simulink model "PARED_RT_SFR"  (R2015a)
settings: Solver=ode4  SolverMode=SingleTasking  StartTime=0.0  StopTime=inf  FixedStep=ts  RelTol=1e-3
InitFcn:
  | tc=ts;
values from neighbouring files (symbols this model uses):
  Kcd = place(matAd,matBud,polosd_lc)    [CONTROL_SEGWAY_BASE_PASADO.m]    (also in analiza_robustez_SFR.m = Kcd.*repmat(Ybase',n_u,1).*repmat(1../Ubase,1,n_y); diseno_control_integral.m = Ka(1, 1:3); diseno_regulador.m = place(Ad, Bd, polosd_lc); maestro.m = place (matAd , matBd , polosd_lc))
  Kcd_pared = acker(matAdp,matBdp(:,1),polosd_lc_pared)    [CONTROL_SEGWAY_BASE_PASADO.m]    (also in diseno_control_seguimiento_pared.m = place(Adp, Bdp(:,1), polosd_lcp))
  Kid = Kad(:,4)    [CONTROL_SEGWAY_BASE_PASADO.m]    (also in diseno_control_integral.m = Ka(1,4))
  R = 81.6e-3/2    (= 0.0408)    [CONTROL_SEGWAY.m]    (also in CONTROL_SEGWAY_BASE_PASADO.m; diseno_control_integral.m; diseno_control_pid.m; diseno_regulador.m)
  sound_freq = 440    [CONTROL_SEGWAY.m]    (also in CONTROL_SEGWAY_BASE_PASADO.m; diseno_control_integral.m; diseno_control_pid.m; diseno_regulador.m)
  time_start = 1    [CONTROL_SEGWAY.m]    (also in CONTROL_SEGWAY_BASE_PASADO.m; diseno_control_integral.m; diseno_control_pid.m; diseno_regulador.m)
  ts = 5e-3    (= 0.005)    [CONTROL_SEGWAY.m]    (also in CONTROL_SEGWAY_BASE_PASADO.m = 0.1; analiza_robustez_SFR.m = Pss_d.Ts; diseno_control_integral.m; diseno_control_pid.m)
  W = 0.15    [CONTROL_SEGWAY.m]    (also in CONTROL_SEGWAY_BASE_PASADO.m; diseno_control_integral.m; diseno_control_pid.m; diseno_regulador.m)
  Wfc = 0.98    [CONTROL_SEGWAY.m]    (also in CONTROL_SEGWAY_BASE_PASADO.m; diseno_control_integral.m; diseno_control_pid.m; diseno_regulador.m)
undefined symbols (not defined in the file or in its folder): D, D1, D2, Fi, gr, mm, rw, th
undefined symbols (not defined in the file): alfa1, gyro0
libraries: legonxtlib x22, simulink x4
settings Model: SimulationMode=external  ExtModeTrigDuration=2  Creator=jrperez  LastModifiedBy=zamora
settings DataIOCC: SignalLoggingSaveFormat=ModelDataLogs
settings OptimizationCC: ExpressionDepthLimit=2147483647  OptimizeModelRefInitCode=on  LifeSpan=1
settings DebuggingCC: UnderspecifiedInitializationDetection=Classic  MergeDetectMultiDrivingBlocksExec=none  ParameterPrecisionLossMsg=none  FcnCallInpInsideContextMsg=EnableAllAsWarning  StateNameClashWarn=warning
settings HardwareCC: ProdLargestAtomicInteger=Long  ProdLargestAtomicFloat=Float  ProdEndianess=LittleEndian  ProdHWDeviceType=ARM Compatible->ARM 7
settings RTWCC: SystemTargetFile=realtime.tlc  GenerateMakefile=off  TemplateMakefile=realtime.tmf  Description=Real-Time Toolbox  RTWVerbose=off
settings CodeAppCC: CustomSymbolStrType=$N$R$M  InternalIdentifier=Classic
settings ERTTargetCC: CombineOutputUpdateFcns=off  ExtMode=on  ExtModeTransport=2  ExtModeMexFile=ext_serial_win32_comm_no_acks_rtt  ExtModeMexArgs=0 10 9600 30  InlinedParameterPlacement=Hierarchical  ERTSrcFileBannerTemplate=realtime_code_template.cgt  ERTHdrFileBannerTemplate=realtime_code_template.cgt  ERTDataSrcFileTemplate=realtime_code_template.cgt  ERTDataHdrFileTemplate=realtime_code_template.cgt  ERTCustomFileTemplate=realtime_file_process.tlc

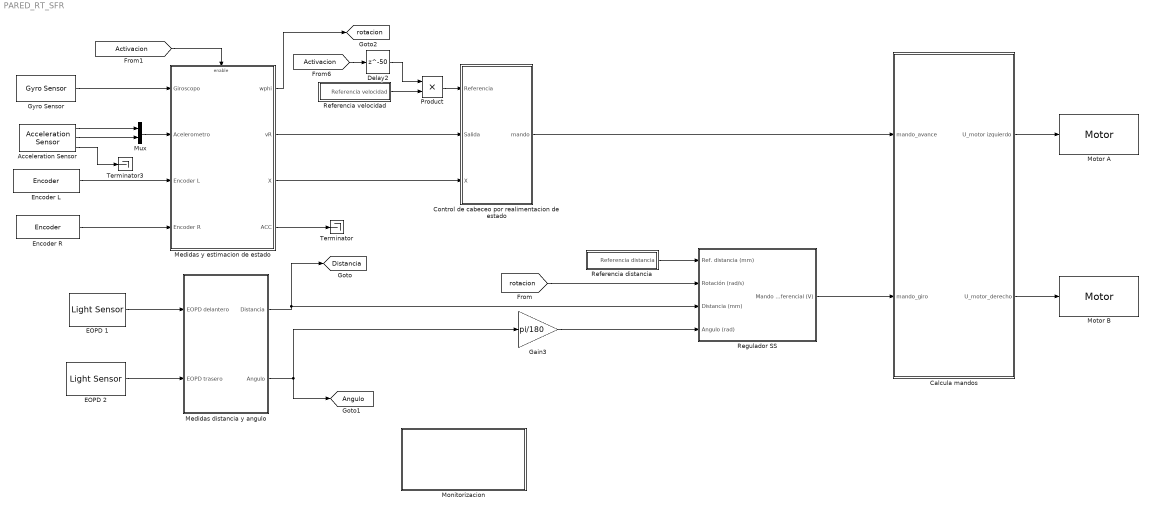
== system PARED_RT_SFR ==
  Acceleration Sensor : legonxtlib/Acceleration Sensor  portNumber=2  sampleTime=ts  blockPlatform=LegoMindstormsNXT
  Calcula mandos : Subsystem
  Control de cabeceo por realimentacion de estado : Subsystem
  Delay2 : Delay  DelayLength=50
  EOPD 1 : legonxtlib/Light Sensor  portNumber=1  outputMode=Raw A/D (1023 - 0)  lightOn=on  sampleTime=ts  blockPlatform=LegoMindstormsNXT
  EOPD 2 : legonxtlib/Light Sensor  portNumber=4  outputMode=Raw A/D (1023 - 0)  lightOn=on  sampleTime=ts  blockPlatform=LegoMindstormsNXT
  Encoder L : legonxtlib/Encoder  portNumber=B  opMode=No reset  sampleTime=ts  blockPlatform=LegoMindstormsNXT
  Encoder R : legonxtlib/Encoder  portNumber=C  opMode=No reset  sampleTime=ts  blockPlatform=LegoMindstormsNXT
  Gain3 : Gain  Gain=pi/180
  Gyro Sensor : legonxtlib/Gyro Sensor  portNumber=3  outputMode=Raw A/D (0 - 1023)  offset=600  sampleTime=ts  blockPlatform=LegoMindstormsNXT
  Medidas distancia y angulo : Subsystem
  Medidas y estimacion de estado : Subsystem
  Monitorizacion : Subsystem
  Motor A : legonxtlib/Motor  sportNumber=B  sstopAction=Brake  blockPlatform=LegoMindstormsNXT
  Motor B : legonxtlib/Motor  sportNumber=C  sstopAction=Brake  blockPlatform=LegoMindstormsNXT
  Mux : Mux  Inputs=2
  Product : Product  RndMeth=Zero
  Referencia distancia : Subsystem
  Referencia velocidad : Subsystem
  Regulador SS : Subsystem
  Terminator : Terminator
  Terminator3 : Terminator
  tag scope: Angulo=global, Distancia=global, rotacion=global
  wires:
  Calcula mandos/1(U_motor izquierdo) -> Motor A/1
  Calcula mandos/2(U_motor_derecho) -> Motor B/1
  Control de cabeceo por realimentacion de estado/1(mando) -> Calcula mandos/1(mando_avance)
  EOPD 1/1 -> Medidas distancia y angulo/1(EOPD delantero)
  EOPD 2/1 -> Medidas distancia y angulo/2(EOPD trasero)
  Medidas distancia y angulo/1(Distancia) -> Regulador SS/3(Distancia (mm)), [Distancia]
  Medidas y estimacion de estado/4(ACC) -> Terminator/1
  [Activacion] -> Delay2/1
  Product/1 -> Control de cabeceo por realimentacion de estado/1(Referencia)
  Referencia velocidad/1(Referencia velocidad) -> Product/2
  Delay2/1 -> Product/1
  Gyro Sensor/1 -> Medidas y estimacion de estado/1(Giroscopo)
  Encoder L/1 -> Medidas y estimacion de estado/3(Encoder L)
  Encoder R/1 -> Medidas y estimacion de estado/4(Encoder R)
  Acceleration Sensor/3 -> Terminator3/1
  Acceleration Sensor/1 -> Mux/1
  Acceleration Sensor/2 -> Mux/2
  Mux/1 -> Medidas y estimacion de estado/2(Acelerometro)
  Medidas y estimacion de estado/2(vR) -> Control de cabeceo por realimentacion de estado/2(Salida)
  Medidas y estimacion de estado/3(X) -> Control de cabeceo por realimentacion de estado/3(X)
  [Activacion] -> Medidas y estimacion de estado/Enable
  Medidas y estimacion de estado/1(wphi) -> [rotacion]
  Medidas distancia y angulo/2(Angulo) -> [Angulo], Gain3/1
  [rotacion] -> Regulador SS/2(Rotación (rad/s))
  Referencia distancia/1(Referencia distancia) -> Regulador SS/1(Ref. distancia (mm))
  Gain3/1 -> Regulador SS/4(Angulo (rad))
  Regulador SS/1(Mando diferencial (V)) -> Calcula mandos/2(mando_giro)

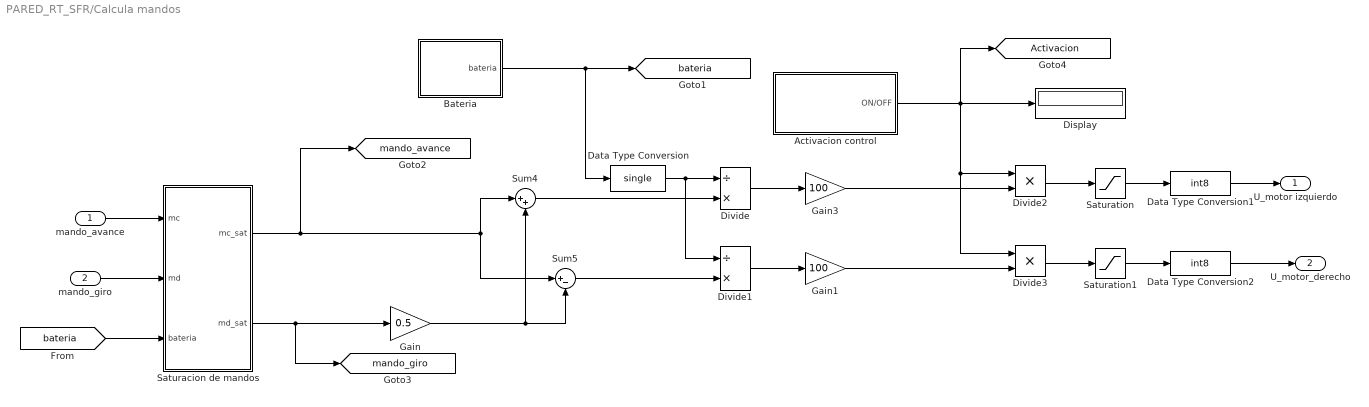
== system PARED_RT_SFR/Calcula mandos ==
  mando_avance : Inport
  mando_giro : Inport  Port=2
  Activacion control : Subsystem
  Bateria : Subsystem
  Data Type Conversion : DataTypeConversion  OutDataTypeStr=single  SampleTime=ts
  Data Type Conversion1 : DataTypeConversion  OutDataTypeStr=int8
  Data Type Conversion2 : DataTypeConversion  OutDataTypeStr=int8
  Display : Display
  Divide : Product  Inputs=/*  SampleTime=ts
  Divide1 : Product  Inputs=/*  SampleTime=ts
  Divide2 : Product  SampleTime=ts
  Divide3 : Product  SampleTime=ts
  Gain : Gain  Gain=0.5  OutDataTypeStr=single
  Gain1 : Gain  Gain=100
  Gain3 : Gain  Gain=100
  Saturacion de mandos : Subsystem
  Saturation : Saturate  UpperLimit=100  LowerLimit=-100
  Saturation1 : Saturate  UpperLimit=100  LowerLimit=-100
  Sum4 : Sum  Inputs=|++
  Sum5 : Sum  Inputs=|+-
  U_motor izquierdo : Outport
  U_motor_derecho : Outport  Port=2
  tag scope: Activacion=global, bateria=global, mando_avance=global, mando_giro=global
  wires:
  Divide/1 -> Gain3/1
  Sum4/1 -> Divide/2
  Gain3/1 -> Divide2/2
  Divide1/1 -> Gain1/1
  Sum5/1 -> Divide1/2
  Saturacion de mandos/1(mc_sat) -> Sum4/1, Sum5/1, [mando_avance]
  Saturacion de mandos/2(md_sat) -> [mando_giro], Gain/1
  Bateria/1(bateria) -> Data Type Conversion/1, [bateria]
  Divide2/1 -> Saturation/1
  Divide3/1 -> Saturation1/1
  Data Type Conversion1/1 -> U_motor izquierdo/1
  Data Type Conversion2/1 -> U_motor_derecho/1
  Data Type Conversion/1 -> Divide/1, Divide1/1
  Gain1/1 -> Divide3/2
  Saturation/1 -> Data Type Conversion1/1
  Saturation1/1 -> Data Type Conversion2/1
  [bateria] -> Saturacion de mandos/3(bateria)
  mando_avance/1 -> Saturacion de mandos/1(mc)
  mando_giro/1 -> Saturacion de mandos/2(md)
  Activacion control/1(ON/OFF) -> Display/1, [Activacion], Divide2/1, Divide3/1
  Gain/1 -> Sum4/2, Sum5/2

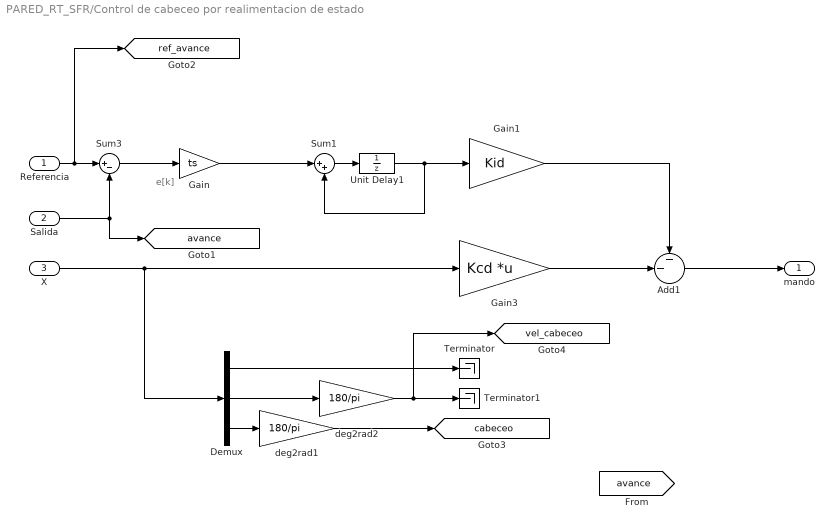
== system PARED_RT_SFR/Control de cabeceo por realimentacion de estado ==
  note: e[k]
  Referencia : Inport
  Salida : Inport  Port=2
  X : Inport  Port=3  SampleTime=ts
  Add1 : Sum  Inputs=--|
  Demux : Demux  Outputs=3
  Gain : Gain  Gain=ts  RndMeth=Simplest  OutDataTypeStr=Inherit: Same as input
  Gain1 : Gain  Gain=Kid  RndMeth=Simplest  SaturateOnIntegerOverflow=on  OutDataTypeStr=Inherit: Same as input  ParamDataTypeStr=Inherit: Same as input
  Gain3 : Gain  Gain=Kcd  Multiplication=Matrix(K*u) (u vector)  SaturateOnIntegerOverflow=on  OutDataTypeStr=Inherit: Same as input  ParamDataTypeStr=Inherit: Same as input
  Sum1 : Sum  Inputs=|++  AccumDataTypeStr=single
  Sum3 : Sum  Inputs=|+-  AccumDataTypeStr=single
  Terminator : Terminator
  Terminator1 : Terminator
  Unit Delay1 : UnitDelay  SampleTime=-1
  deg2rad1 : Gain  Gain=180/pi  OutDataTypeStr=Inherit: Same as input  ParamDataTypeStr=Inherit: Same as input
  deg2rad2 : Gain  Gain=180/pi  OutDataTypeStr=Inherit: Same as input  ParamDataTypeStr=Inherit: Same as input
  mando : Outport
  tag scope: avance=global, cabeceo=global, ref_avance=global, vel_cabeceo=global
  wires:
  Add1/1 -> mando/1
  Unit Delay1/1 -> Gain1/1, Sum1/2
  Referencia/1 -> Sum3/1, [ref_avance]
  Salida/1 -> Sum3/2, [avance]
  Sum3/1 -> Gain/1
  Sum1/1 -> Unit Delay1/1
  Gain1/1 -> Add1/1
  Gain3/1 -> Add1/2
  X/1 -> Gain3/1, Demux/1
  Demux/1 -> Terminator/1
  Demux/2 -> deg2rad2/1
  Demux/3 -> deg2rad1/1
  deg2rad1/1 -> [cabeceo]
  Gain/1 -> Sum1/1
  deg2rad2/1 -> [vel_cabeceo], Terminator1/1

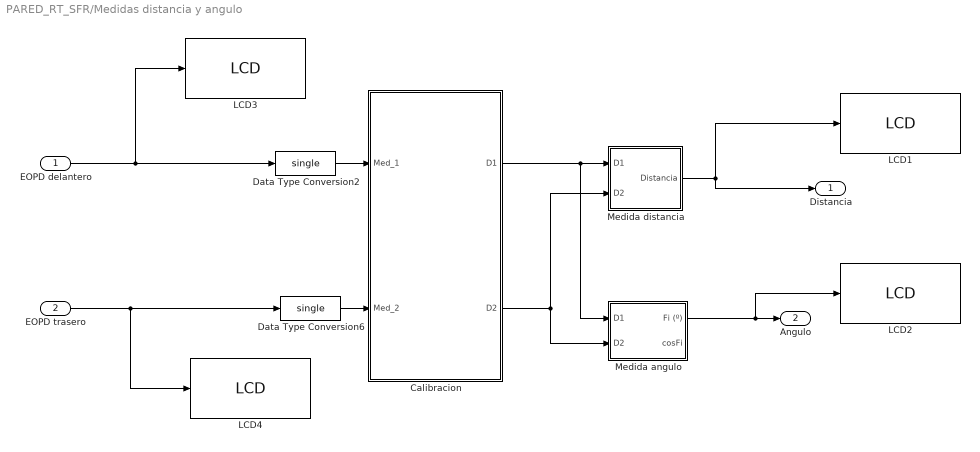
== system PARED_RT_SFR/Medidas distancia y angulo ==
  EOPD delantero : Inport
  EOPD trasero : Inport  Port=2
  "Calibracion " : Subsystem  mask{distNear=50, distFar=100, eopdNear_1=725, eopdNear_2=732, eopdFar_1=917, eopdFar_2=922, ts=ts}
      mask prompts: distNear "Distancia cercana (mm)"; distFar "Distancia lejana (mm)"; eopdNear_1 "Medida D1 cercana (raw)"; eopdNear_2 "Medida D2  cercana (raw)"; eopdFar_1 "Medida D1 lejana (raw)"; eopdFar_2 "Medida D2 lejana (raw)"; ts "Período de muestreo"
      mask init:
      | % Ver justificacion en:
      | % http://www.hitechnic.com/blog/eopd-sensor/eopd-how-to-measure-distance/
  Data Type Conversion2 : DataTypeConversion  OutDataTypeStr=single
  Data Type Conversion6 : DataTypeConversion  OutDataTypeStr=single
  LCD1 : legonxtlib/LCD  slcdStr=D(mm)  slcdLine=1  slcdFormat=Decimal  blockPlatform=LegoMindstormsNXT
  LCD2 : legonxtlib/LCD  slcdStr=Fi(gr)  slcdLine=2  slcdFormat=Decimal  blockPlatform=LegoMindstormsNXT
  LCD3 : legonxtlib/LCD  slcdStr=D1(rw)  slcdLine=3  slcdFormat=Decimal  blockPlatform=LegoMindstormsNXT
  LCD4 : legonxtlib/LCD  slcdStr=D2(rw)  slcdLine=4  slcdFormat=Decimal  blockPlatform=LegoMindstormsNXT
  Medida distancia : Subsystem
  Medida angulo : Subsystem
  Distancia : Outport
  Angulo : Outport  Port=2
  wires:
  Data Type Conversion2/1 -> "Calibracion "/1(Med_1)
  Data Type Conversion6/1 -> "Calibracion "/2(Med_2)
  EOPD delantero/1 -> Data Type Conversion2/1, LCD3/1
  EOPD trasero/1 -> Data Type Conversion6/1, LCD4/1
  "Calibracion "/1(D1) -> Medida distancia/1(D1), Medida angulo/1(D1)
  "Calibracion "/2(D2) -> Medida distancia/2(D2), Medida angulo/2(D2)
  Medida angulo/1(Fi (º)) -> Angulo/1, LCD2/1
  Medida distancia/1(Distancia) -> Distancia/1, LCD1/1

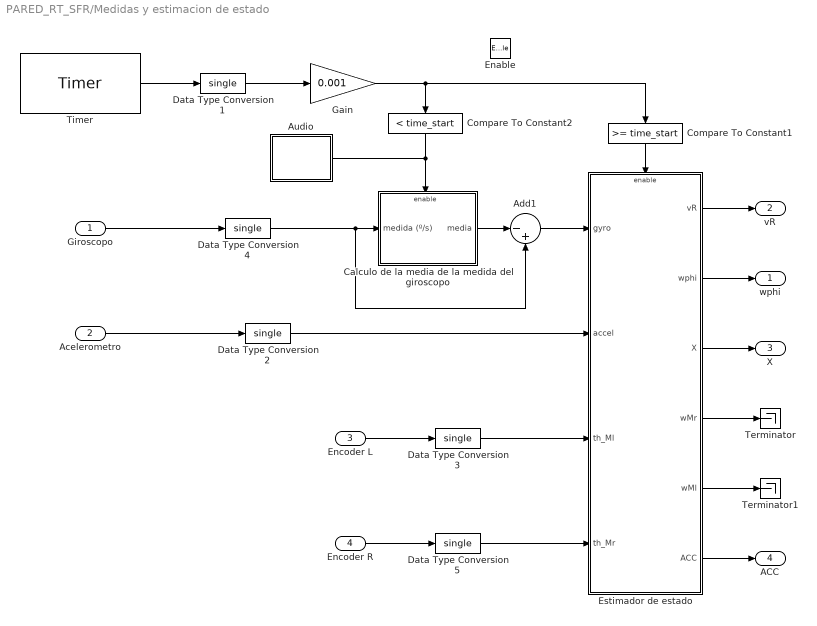
== system PARED_RT_SFR/Medidas y estimacion de estado ==
  Giroscopo : Inport
  Acelerometro : Inport  Port=2
  Encoder L : Inport  Port=3
  Encoder R : Inport  Port=4
  Enable : EnablePort
  Add1 : Sum  Inputs=|-+
  Audio : Subsystem
  Calculo de la media de la medida del giroscopo : Subsystem
  Compare To Constant1 : simulink/Logic and Bit Operations/Compare To Constant  relop=>=  const=time_start  OutDataTypeStr=boolean
  Compare To Constant2 : simulink/Logic and Bit Operations/Compare To Constant  relop=<  const=time_start  OutDataTypeStr=boolean
  Data Type Conversion{1..5} (5 alike) : DataTypeConversion  OutDataTypeStr=single  RndMeth=Simplest
      settings: AttributesFormatString=Round = %<RndMeth>
  Estimador de estado : Subsystem
  Gain : Gain  Gain=0.001
  Terminator : Terminator
  Terminator1 : Terminator
  Timer : legonxtlib/Timer  sampleTime=ts  blockPlatform=LegoMindstormsNXT
  wphi : Outport
  vR : Outport  Port=2
  X : Outport  Port=3
  ACC : Outport  Port=4
  wires:
  Data Type Conversion4/1 -> Calculo de la media de la medida del giroscopo/1(medida (º/s)), Add1/2
  Calculo de la media de la medida del giroscopo/1(media) -> Add1/1
  Giroscopo/1 -> Data Type Conversion4/1
  Compare To Constant2/1 -> Calculo de la media de la medida del giroscopo/Enable, Audio/Enable
  Encoder L/1 -> Data Type Conversion3/1
  Encoder R/1 -> Data Type Conversion5/1
  Add1/1 -> Estimador de estado/1(gyro)
  Data Type Conversion3/1 -> Estimador de estado/3(th_Ml)
  Data Type Conversion5/1 -> Estimador de estado/4(th_Mr)
  Estimador de estado/5(wMl) -> Terminator1/1
  Estimador de estado/4(wMr) -> Terminator/1
  Estimador de estado/1(vR) -> vR/1
  Estimador de estado/2(wphi) -> wphi/1
  Estimador de estado/3(X) -> X/1
  Gain/1 -> Compare To Constant2/1, Compare To Constant1/1
  Timer/1 -> Data Type Conversion1/1
  Compare To Constant1/1 -> Estimador de estado/Enable
  Data Type Conversion1/1 -> Gain/1
  Data Type Conversion2/1 -> Estimador de estado/2(accel)
  Acelerometro/1 -> Data Type Conversion2/1
  Estimador de estado/6(ACC) -> ACC/1

== system PARED_RT_SFR/Monitorizacion ==
  Medidas : Scope
      settings: TimeRange=auto  MaxDataPoints=5000  SaveName=Medidas  YMin=-10  YMax=10  SampleTime=-1  DataFormat=Array
  Mux1 : Mux  Inputs=8
  wires:
  Mux1/1 -> Medidas/1
  [cabeceo] -> Mux1/1
  [vel_cabeceo] -> Mux1/2
  [avance] -> Mux1/3
  [mando_avance] -> Mux1/4
  [Distancia] -> Mux1/5
  [rotacion] -> Mux1/7
  [Angulo] -> Mux1/6
  [mando_giro] -> Mux1/8

== system PARED_RT_SFR/Referencia distancia ==
  ang_ref maximo2 : Constant  Value=100  OutDataTypeStr=single  SampleTime=ts
  Referencia distancia : Outport
  wires:
  ang_ref maximo2/1 -> Referencia distancia/1

== system PARED_RT_SFR/Referencia velocidad ==
  ang_ref maximo2 : Constant  Value=-0.15  OutDataTypeStr=single  SampleTime=ts
  Referencia velocidad : Outport
  wires:
  ang_ref maximo2/1 -> Referencia velocidad/1

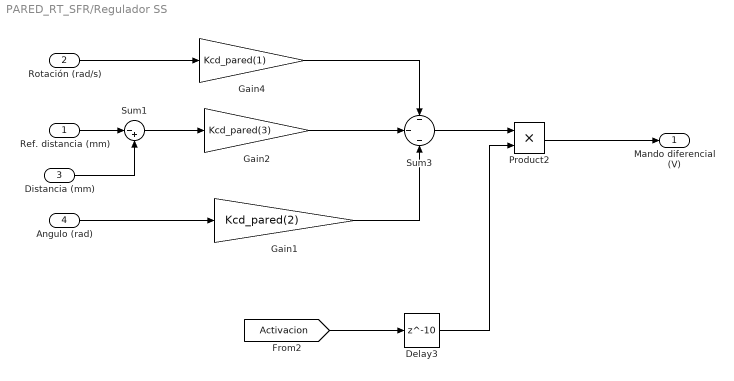
== system PARED_RT_SFR/Regulador SS ==
  Ref. distancia (mm) : Inport
  Rotación (rad/s) : Inport  Port=2
  Distancia (mm) : Inport  Port=3
  Angulo (rad) : Inport  Port=4
  Delay3 : Delay  DelayLength=10
  Gain1 : Gain  Gain=Kcd_pared(2)
  Gain2 : Gain  Gain=Kcd_pared(3)
  Gain4 : Gain  Gain=Kcd_pared(1)
  Product2 : Product  RndMeth=Zero
  Sum1 : Sum  Inputs=|-+
  Sum3 : Sum  Inputs=-|-|-
  Mando diferencial (V) : Outport
  wires:
  Sum1/1 -> Gain2/1
  Sum3/1 -> Product2/1
  Delay3/1 -> Product2/2
  Gain1/1 -> Sum3/3
  Gain4/1 -> Sum3/1
  Rotación (rad/s)/1 -> Gain4/1
  Angulo (rad)/1 -> Gain1/1
  Product2/1 -> Mando diferencial (V)/1
  [Activacion] -> Delay3/1
  Ref. distancia (mm)/1 -> Sum1/1
  Gain2/1 -> Sum3/2
  Distancia (mm)/1 -> Sum1/2

== system PARED_RT_SFR/Calcula mandos/Activacion control ==
  Button : legonxtlib/Button  buttonType=Middle orange  sampleTime=0.1  blockPlatform=LegoMindstormsNXT
  Data Type Conversion : DataTypeConversion  OutDataTypeStr=single
  Saturation : Saturate  UpperLimit=1  LowerLimit=0
  Switch : Switch  Threshold=0.5
  Unit Delay : UnitDelay  SampleTime=0.1
  ON/OFF : Outport
  wires:
  Button/1 -> Data Type Conversion/1
  Switch/1 -> Saturation/1
  Unit Delay/1 -> Switch/3
  Data Type Conversion/1 -> Switch/2, Switch/1
  Saturation/1 -> Unit Delay/1, ON/OFF/1

== system PARED_RT_SFR/Calcula mandos/Bateria ==
  Battery : legonxtlib/Battery  sampleTime=0.1  blockPlatform=LegoMindstormsNXT
  Data Type Conversion : DataTypeConversion  OutDataTypeStr=double
  Data Type Conversion1 : DataTypeConversion  OutDataTypeStr=single
  Gain1 : Gain  Gain=1/5
  Gain6 : Gain  Gain=0.001
  Integrator : Integrator  InitialConditionSource=external
  Sum1 : Sum  Inputs=|+-
  bateria : Outport
  wires:
  Battery/1 -> Data Type Conversion/1
  Data Type Conversion/1 -> Gain6/1
  Sum1/1 -> Gain1/1
  Integrator/1 -> Sum1/2, Data Type Conversion1/1
  Gain6/1 -> Sum1/1, Integrator/2
  Gain1/1 -> Integrator/1
  Data Type Conversion1/1 -> bateria/1

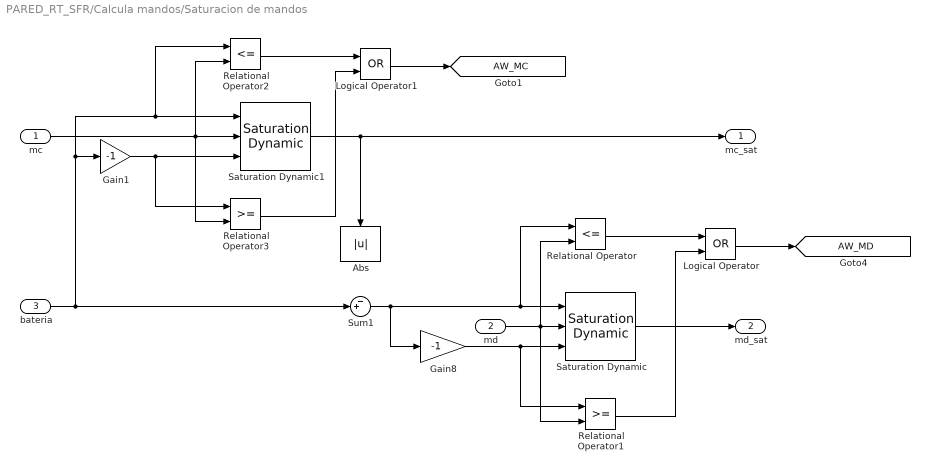
== system PARED_RT_SFR/Calcula mandos/Saturacion de mandos ==
  mc : Inport
  md : Inport  Port=2
  bateria : Inport  Port=3  SampleTime=ts
  Abs : Abs
  Gain1 : Gain  Gain=-1
  Gain8 : Gain  Gain=-1
  Logical Operator : Logic  Operator=OR  AllPortsSameDT=off  OutDataTypeStr=boolean
  Logical Operator1 : Logic  Operator=OR  AllPortsSameDT=off  OutDataTypeStr=boolean
  Relational Operator : RelationalOperator  Operator=<=  OutDataTypeStr=boolean
  Relational Operator1 : RelationalOperator  OutDataTypeStr=boolean
  Relational Operator2 : RelationalOperator  Operator=<=  OutDataTypeStr=boolean
  Relational Operator3 : RelationalOperator  OutDataTypeStr=boolean
  Saturation Dynamic : simulink/Discontinuities/Saturation Dynamic  OutMin=[]  OutMax=[]  OutDataTypeStr=Inherit: Same as second input  OutDataType=fixdt(1, 16)  OutScaling=2^-10  DoSatur=off
  Saturation Dynamic1 : simulink/Discontinuities/Saturation Dynamic  OutMin=[]  OutMax=[]  OutDataTypeStr=Inherit: Same as second input  OutDataType=fixdt(1, 16)  OutScaling=2^-10  DoSatur=off
  Sum1 : Sum  Inputs=-+|
  mc_sat : Outport
  md_sat : Outport  Port=2
  tag scope: AW_MC=global, AW_MD=global
  wires:
  Saturation Dynamic1/1 -> Abs/1, mc_sat/1
  Gain8/1 -> Saturation Dynamic/3, Relational Operator1/1
  Sum1/1 -> Gain8/1, Saturation Dynamic/1, Relational Operator/1
  mc/1 -> Saturation Dynamic1/2, Relational Operator2/2, Relational Operator3/2
  md/1 -> Saturation Dynamic/2, Relational Operator/2, Relational Operator1/2
  Saturation Dynamic/1 -> md_sat/1
  bateria/1 -> Sum1/2, Gain1/1, Saturation Dynamic1/1, Relational Operator2/1
  Relational Operator/1 -> Logical Operator/1
  Relational Operator1/1 -> Logical Operator/2
  Logical Operator/1 -> [AW_MD]
  Gain1/1 -> Saturation Dynamic1/3, Relational Operator3/1
  Relational Operator2/1 -> Logical Operator1/1
  Logical Operator1/1 -> [AW_MC]
  Relational Operator3/1 -> Logical Operator1/2

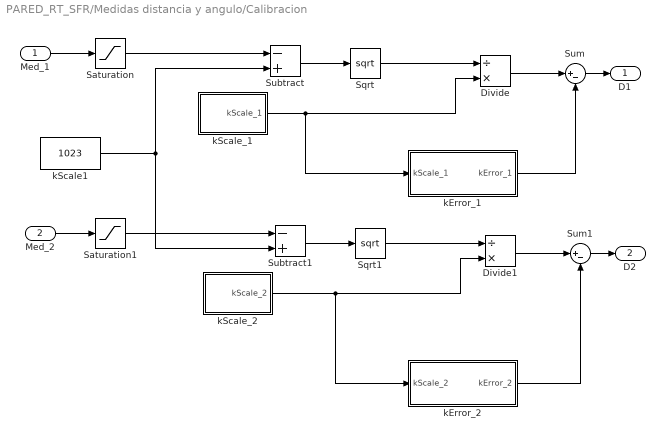
== system PARED_RT_SFR/Medidas distancia y angulo/Calibracion  ==
  Med_1 : Inport
  Med_2 : Inport  Port=2
  Divide : Product  Inputs=/*
  Divide1 : Product  Inputs=/*
  Saturation : Saturate  UpperLimit=1022  LowerLimit=1
  Saturation1 : Saturate  UpperLimit=1022  LowerLimit=1
  Sqrt : Sqrt  SaturateOnIntegerOverflow=on
  Sqrt1 : Sqrt  SaturateOnIntegerOverflow=on
  Subtract : Sum  Inputs=-+
  Subtract1 : Sum  Inputs=-+
  Sum : Sum  Inputs=|+-
  Sum1 : Sum  Inputs=|+-
  kError_1 : Subsystem
  kError_2 : Subsystem
  kScale1 : Constant  Value=1023  OutDataTypeStr=single  SampleTime=ts
  kScale_1 : Subsystem
  kScale_2 : Subsystem
  D1 : Outport
  D2 : Outport  Port=2
  wires:
  Sqrt/1 -> Divide/1
  kScale_1/1(kScale_1) -> kError_1/1(kScale_1), Divide/2
  Divide/1 -> Sum/1
  kError_1/1(kError_1) -> Sum/2
  Med_1/1 -> Saturation/1
  Sum/1 -> D1/1
  Sqrt1/1 -> Divide1/1
  kScale_2/1(kScale_2) -> Divide1/2, kError_2/1(kScale_2)
  Divide1/1 -> Sum1/1
  kError_2/1(kError_2) -> Sum1/2
  Med_2/1 -> Saturation1/1
  Sum1/1 -> D2/1
  Subtract1/1 -> Sqrt1/1
  Subtract/1 -> Sqrt/1
  kScale1/1 -> Subtract/2, Subtract1/2
  Saturation/1 -> Subtract/1
  Saturation1/1 -> Subtract1/1

== system PARED_RT_SFR/Medidas distancia y angulo/Medida distancia ==
  D1 : Inport
  D2 : Inport  Port=2
  Gain3 : Gain  Gain=1/2
  Sum6 : Sum  Inputs=|++
  Distancia : Outport
  wires:
  Gain3/1 -> Distancia/1
  D2/1 -> Sum6/2
  Sum6/1 -> Gain3/1
  D1/1 -> Sum6/1

== system PARED_RT_SFR/Medidas distancia y angulo/Medida angulo ==
  D1 : Inport
  D2 : Inport  Port=2
  D3 : Constant  Value=120  OutDataTypeStr=single
  Divide2 : Product  Inputs=*/
  Gain3 : Gain  Gain=180/pi
  Sum3 : Sum  Inputs=|+-
  Trigonometric Function1 : Trigonometry  Operator=atan
  Trigonometric Function2 : Trigonometry  Operator=cos
  Fi (º) : Outport
  cosFi : Outport  Port=2
  wires:
  Trigonometric Function1/1 -> Gain3/1, Trigonometric Function2/1
  D1/1 -> Sum3/1
  Gain3/1 -> Fi (º)/1
  D2/1 -> Sum3/2
  Trigonometric Function2/1 -> cosFi/1
  Divide2/1 -> Trigonometric Function1/1
  Sum3/1 -> Divide2/1
  D3/1 -> Divide2/2

== system PARED_RT_SFR/Medidas y estimacion de estado/Audio ==
  Enable : EnablePort
  Constant2 : Constant  Value=sound_freq  OutDataTypeStr=single  SampleTime=0.2
      settings: AttributesFormatString=DataType = %<OutDataTypeStr>
  Speaker : legonxtlib/Speaker  sinputMode=Frequency only  sspeakerFreq=100  sspeakerVolume=50  sspeakerDuration=100  blockPlatform=LegoMindstormsNXT
  wires:
  Constant2/1 -> Speaker/1

== system PARED_RT_SFR/Medidas y estimacion de estado/Calculo de la media de la medida del giroscopo ==
  medida (º/s) : Inport  SampleTime=ts
  Enable : EnablePort
  Filtro digital paso bajo : Subsystem  mask{alfa=alfa1, x0=gyro0, ts=ts}
      mask prompts: alfa "Constante de filtrado"; x0 "Condición inicial"; ts "Período de muestreo"
  media : Outport
  wires:
  medida (º/s)/1 -> Filtro digital paso bajo/1(ent)
  Filtro digital paso bajo/1(sal) -> media/1

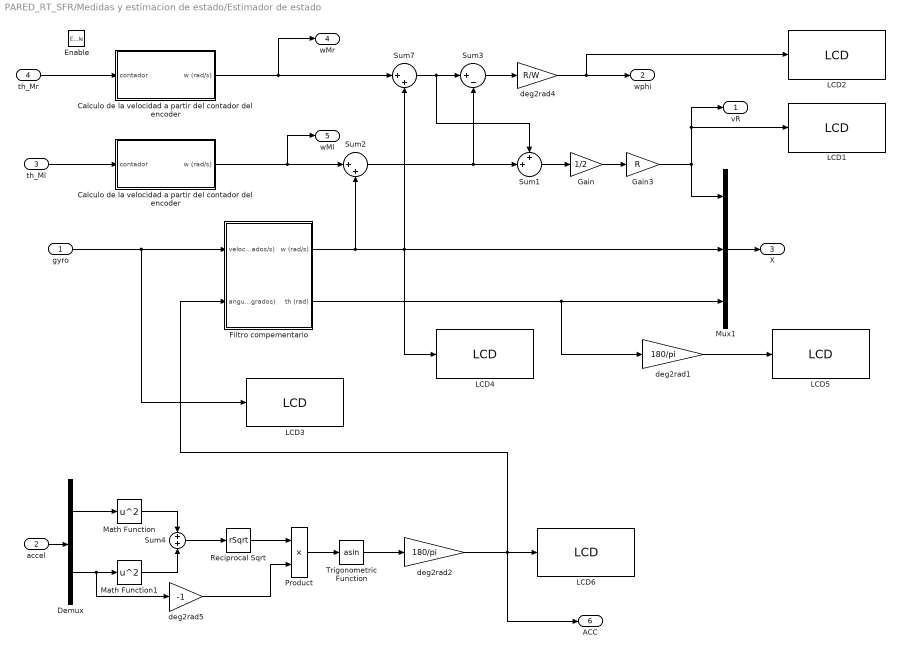
== system PARED_RT_SFR/Medidas y estimacion de estado/Estimador de estado ==
  gyro : Inport
  accel : Inport  Port=2
  th_Ml : Inport  Port=3
  th_Mr : Inport  Port=4
  Enable : EnablePort
  Calculo de la velocidad a partir del contador del encoder : Subsystem  mask{GpT=1, alfa=alfa1, ts=ts}
      mask prompts: GpT "grados/tick"; alfa "Constante de filtrado paso bajo"; ts "Período de muestreo"
  "Calculo de la velocidad a partir del contador del encoder " : Subsystem  mask{GpT=1, alfa=alfa1, ts=ts}
      mask prompts: GpT "grados/tick"; alfa "Constante de filtrado paso bajo"; ts "Período de muestreo"
  Demux : Demux  Outputs=2
  Filtro compementario : Subsystem
  Gain : Gain  Gain=1/2  OutDataTypeStr=Inherit: Same as input  ParamDataTypeStr=Inherit: Same as input
  Gain3 : Gain  Gain=R  OutDataTypeStr=Inherit: Same as input  ParamDataTypeStr=Inherit: Same as input
  LCD1 : legonxtlib/LCD  slcdStr=vR  slcdLine=1  slcdFormat=Decimal  blockPlatform=LegoMindstormsNXT
  LCD2 : legonxtlib/LCD  slcdStr=wphi  slcdLine=2  slcdFormat=Decimal  blockPlatform=LegoMindstormsNXT
  LCD3 : legonxtlib/LCD  slcdStr=gyro  slcdLine=3  slcdFormat=Decimal  blockPlatform=LegoMindstormsNXT
  LCD4 : legonxtlib/LCD  slcdStr=wth  slcdLine=4  slcdFormat=Decimal  blockPlatform=LegoMindstormsNXT
  LCD5 : legonxtlib/LCD  slcdStr=th (º)  slcdLine=5  slcdFormat=Decimal  blockPlatform=LegoMindstormsNXT
  LCD6 : legonxtlib/LCD  slcdStr=th(º)  slcdLine=6  slcdFormat=Decimal  blockPlatform=LegoMindstormsNXT
  Math Function : Math  Operator=square  SaturateOnIntegerOverflow=on
  Math Function1 : Math  Operator=square  SaturateOnIntegerOverflow=on
  Mux1 : Mux  Inputs=3
  Product : Product
  Reciprocal Sqrt : Sqrt  Operator=rSqrt  SaturateOnIntegerOverflow=on
  Sum1 : Sum  Inputs=++|  OutDataTypeStr=Inherit: Same as first input
  Sum2 : Sum  Inputs=|++  OutDataTypeStr=Inherit: Same as first input
  Sum3 : Sum  Inputs=|+-
  Sum4 : Sum  Inputs=+|+
  Sum7 : Sum  Inputs=|++
  Trigonometric Function : Trigonometry  Operator=asin
  deg2rad1 : Gain  Gain=180/pi  OutDataTypeStr=Inherit: Same as input  ParamDataTypeStr=Inherit: Same as input
  deg2rad2 : Gain  Gain=180/pi  OutDataTypeStr=Inherit: Same as input  ParamDataTypeStr=Inherit: Same as input
  deg2rad4 : Gain  Gain=R/W  OutDataTypeStr=Inherit: Same as input  ParamDataTypeStr=Inherit: Same as input
  deg2rad5 : Gain  Gain=-1  OutDataTypeStr=Inherit: Same as input  ParamDataTypeStr=Inherit: Same as input
  vR : Outport
  wphi : Outport  Port=2
  X : Outport  Port=3
  wMr : Outport  Port=4
  wMl : Outport  Port=5
  ACC : Outport  Port=6
  wires:
  gyro/1 -> LCD3/1, Filtro compementario/1(velocidad (grados/s))
  Sum2/1 -> Sum1/2, Sum3/2
  Sum7/1 -> Sum1/1, Sum3/1
  Sum3/1 -> deg2rad4/1
  Calculo de la velocidad a partir del contador del encoder/1(w (rad/s)) -> Sum2/1, wMl/1
  "Calculo de la velocidad a partir del contador del encoder "/1(w (rad/s)) -> Sum7/1, wMr/1
  Sum1/1 -> Gain/1
  Mux1/1 -> X/1
  th_Ml/1 -> Calculo de la velocidad a partir del contador del encoder/1(contador)
  th_Mr/1 -> "Calculo de la velocidad a partir del contador del encoder "/1(contador)
  deg2rad4/1 -> wphi/1, LCD2/1
  Gain3/1 -> Mux1/1, LCD1/1, vR/1
  Gain/1 -> Gain3/1
  Filtro compementario/1(w (rad/s)) -> Sum7/2, Mux1/2, LCD4/1, Sum2/2
  Filtro compementario/2(th (rad)) -> Mux1/3, deg2rad1/1
  deg2rad1/1 -> LCD5/1
  Trigonometric Function/1 -> deg2rad2/1
  deg2rad2/1 -> ACC/1, Filtro compementario/2(angulo (grados)), LCD6/1
  accel/1 -> Demux/1
  Demux/1 -> Math Function/1
  Math Function/1 -> Sum4/1
  Math Function1/1 -> Sum4/2
  Sum4/1 -> Reciprocal Sqrt/1
  Reciprocal Sqrt/1 -> Product/1
  Demux/2 -> deg2rad5/1, Math Function1/1
  deg2rad5/1 -> Product/2
  Product/1 -> Trigonometric Function/1

== system PARED_RT_SFR/Medidas distancia y angulo/Calibracion /kError_1 ==
  kScale_1 : Inport
  Divide2 : Product  Inputs=*/
  Sqrt : Sqrt  SaturateOnIntegerOverflow=on
  Subtract2 : Sum  Inputs=+-
  Subtract3 : Sum  Inputs=-+
  disNear : Constant  Value=distNear  OutDataTypeStr=single  SampleTime=ts
  kScale1 : Constant  Value=1023  OutDataTypeStr=single  SampleTime=ts
  kScale4 : Constant  Value=eopdNear_1  OutDataTypeStr=single  SampleTime=ts
  kError_1 : Outport
  wires:
  disNear/1 -> Subtract2/2
  Subtract2/1 -> kError_1/1
  Divide2/1 -> Subtract2/1
  Sqrt/1 -> Divide2/2
  kScale_1/1 -> Divide2/1
  Subtract3/1 -> Sqrt/1
  kScale4/1 -> Subtract3/1
  kScale1/1 -> Subtract3/2

== system PARED_RT_SFR/Medidas distancia y angulo/Calibracion /kError_2 ==
  kScale_2 : Inport
  Divide2 : Product  Inputs=*/
  Sqrt : Sqrt  SaturateOnIntegerOverflow=on
  Subtract2 : Sum  Inputs=+-
  Subtract3 : Sum  Inputs=-+
  disNear1 : Constant  Value=distNear  OutDataTypeStr=single  SampleTime=ts
  kScale1 : Constant  Value=1023  OutDataTypeStr=single  SampleTime=ts
  kScale4 : Constant  Value=eopdNear_2  OutDataTypeStr=single  SampleTime=ts
  kError_2 : Outport
  wires:
  kScale_2/1 -> Divide2/1
  Sqrt/1 -> Divide2/2
  Divide2/1 -> Subtract2/1
  Subtract2/1 -> kError_2/1
  disNear1/1 -> Subtract2/2
  kScale4/1 -> Subtract3/1
  kScale1/1 -> Subtract3/2
  Subtract3/1 -> Sqrt/1

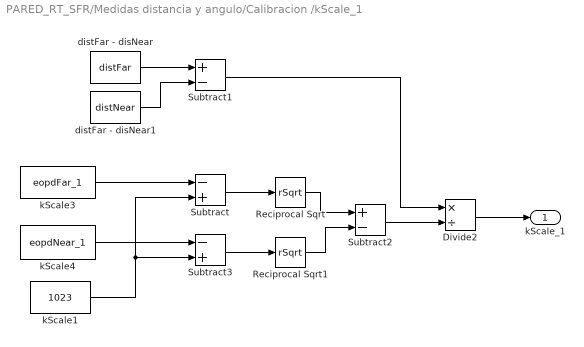
== system PARED_RT_SFR/Medidas distancia y angulo/Calibracion /kScale_1 ==
  Divide2 : Product  Inputs=*/
  Reciprocal Sqrt : Sqrt  Operator=rSqrt  SaturateOnIntegerOverflow=on
  Reciprocal Sqrt1 : Sqrt  Operator=rSqrt  SaturateOnIntegerOverflow=on
  Subtract : Sum  Inputs=-+
  Subtract1 : Sum  Inputs=+-
  Subtract2 : Sum  Inputs=+-
  Subtract3 : Sum  Inputs=-+
  distFar - disNear : Constant  Value=distFar  OutDataTypeStr=single  SampleTime=ts
  distFar - disNear1 : Constant  Value=distNear  OutDataTypeStr=single  SampleTime=ts
  kScale1 : Constant  Value=1023  OutDataTypeStr=single  SampleTime=ts
  kScale3 : Constant  Value=eopdFar_1  OutDataTypeStr=single  SampleTime=ts
  kScale4 : Constant  Value=eopdNear_1  OutDataTypeStr=single  SampleTime=ts
  kScale_1 : Outport
  wires:
  Reciprocal Sqrt/1 -> Subtract2/1
  Reciprocal Sqrt1/1 -> Subtract2/2
  Subtract2/1 -> Divide2/2
  Divide2/1 -> kScale_1/1
  Subtract1/1 -> Divide2/1
  distFar - disNear/1 -> Subtract1/1
  distFar - disNear1/1 -> Subtract1/2
  Subtract/1 -> Reciprocal Sqrt/1
  kScale3/1 -> Subtract/1
  Subtract3/1 -> Reciprocal Sqrt1/1
  kScale4/1 -> Subtract3/1
  kScale1/1 -> Subtract3/2, Subtract/2

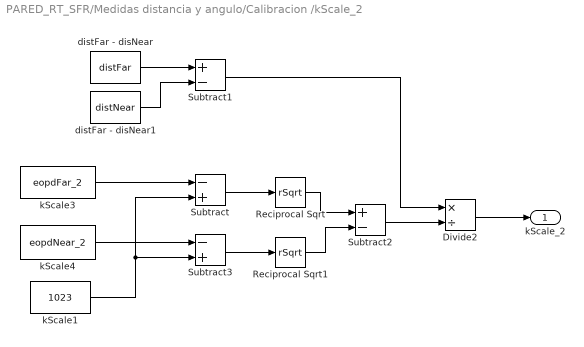
== system PARED_RT_SFR/Medidas distancia y angulo/Calibracion /kScale_2 ==
  Divide2 : Product  Inputs=*/
  Reciprocal Sqrt : Sqrt  Operator=rSqrt  SaturateOnIntegerOverflow=on
  Reciprocal Sqrt1 : Sqrt  Operator=rSqrt  SaturateOnIntegerOverflow=on
  Subtract : Sum  Inputs=-+
  Subtract1 : Sum  Inputs=+-
  Subtract2 : Sum  Inputs=+-
  Subtract3 : Sum  Inputs=-+
  distFar - disNear : Constant  Value=distFar  OutDataTypeStr=single  SampleTime=ts
  distFar - disNear1 : Constant  Value=distNear  OutDataTypeStr=single  SampleTime=ts
  kScale1 : Constant  Value=1023  OutDataTypeStr=single  SampleTime=ts
  kScale3 : Constant  Value=eopdFar_2  OutDataTypeStr=single  SampleTime=ts
  kScale4 : Constant  Value=eopdNear_2  OutDataTypeStr=single  SampleTime=ts
  kScale_2 : Outport
  wires:
  kScale1/1 -> Subtract/2, Subtract3/2
  kScale4/1 -> Subtract3/1
  Subtract3/1 -> Reciprocal Sqrt1/1
  kScale3/1 -> Subtract/1
  Subtract/1 -> Reciprocal Sqrt/1
  distFar - disNear1/1 -> Subtract1/2
  distFar - disNear/1 -> Subtract1/1
  Subtract1/1 -> Divide2/1
  Divide2/1 -> kScale_2/1
  Subtract2/1 -> Divide2/2
  Reciprocal Sqrt1/1 -> Subtract2/2
  Reciprocal Sqrt/1 -> Subtract2/1

== system PARED_RT_SFR/Medidas y estimacion de estado/Calculo de la media de la medida del giroscopo/Filtro digital paso bajo ==
  note: Función de transferencia del filtro
      |                        1-alfa
      |                  ----------------
      |                   1-alfa*z^(-1)
  ent : Inport  SampleTime=ts
  Gain2 : Gain  Gain=alfa  OutDataTypeStr=Inherit: Same as input  ParamDataTypeStr=Inherit: Same as input
  Gain3 : Gain  Gain=1-alfa  OutDataTypeStr=Inherit: Same as input  ParamDataTypeStr=Inherit: Same as input
  Sum : Sum  Inputs=|++  OutDataTypeStr=Inherit: Same as first input
  Unit Delay : UnitDelay  InitialCondition=x0  SampleTime=-1
  sal : Outport
  wires:
  ent/1 -> Gain3/1
  Gain3/1 -> Sum/1
  Gain2/1 -> Sum/2
  Unit Delay/1 -> Gain2/1
  Sum/1 -> sal/1, Unit Delay/1

== system PARED_RT_SFR/Medidas y estimacion de estado/Estimador de estado/Calculo de la velocidad a partir del contador del encoder ==
  contador : Inport  SampleTime=ts
  Derivada discreta : Subsystem  mask{ts=ts, opcion=Derivada en adelanto s=(1-z^-1)/ts}
      mask prompts: ts "Período de muestreo"; opcion "Método de discretización"
      mask init:
      | z=tf('z',ts);
      | switch(opcion)
      |     case 1
      |         derivada=minreal((1-z^-1)/ts);
      |     case 2
      |         derivada=minreal(2*(1-z^-1)/ts/(1+z^-1));
      |     case 3
      |         derivada=minreal((1.5-2*z^-1+0.5*z^-2)/ts);
      | end
      mask TypeOptions opcion: Derivada en adelanto s=(1-z^-1)/ts  | Trapezoidal s=2*(1-z^-1)/ts/(1+z^-1) | Derivada por aproximación parabólica s=(1.5-2*z^-1+0.5z^-2)/ts
  Filtro digital paso bajo : Subsystem  mask{alfa=alfa, x0=0, ts=ts}
      mask prompts: alfa "Constante de filtrado"; x0 "Condición inicial"; ts "Período de muestreo"
  Paso a grados : Gain  Gain=GpT
  Paso a rad/s : Gain  Gain=pi/180
  w (rad/s) : Outport
  wires:
  contador/1 -> Paso a grados/1
  Paso a grados/1 -> Paso a rad/s/1
  Paso a rad/s/1 -> Filtro digital paso bajo/1(ent)
  Filtro digital paso bajo/1(sal) -> Derivada discreta/1(ent)
  Derivada discreta/1(sal) -> w (rad/s)/1

== system PARED_RT_SFR/Medidas y estimacion de estado/Estimador de estado/Calculo de la velocidad a partir del contador del encoder  ==
  contador : Inport  SampleTime=ts
  Derivada discreta : Subsystem  mask{ts=ts, opcion=Derivada en adelanto s=(1-z^-1)/ts}
      mask prompts: ts "Período de muestreo"; opcion "Método de discretización"
      mask init: same as PARED_RT_SFR/Medidas y estimacion de estado/Estimador de estado/Calculo de la velocidad a partir del contador del encoder/Derivada discreta
      mask TypeOptions opcion: Derivada en adelanto s=(1-z^-1)/ts  | Trapezoidal s=2*(1-z^-1)/ts/(1+z^-1) | Derivada por aproximación parabólica s=(1.5-2*z^-1+0.5z^-2)/ts
  Filtro digital paso bajo : Subsystem  mask{alfa=alfa, x0=0, ts=ts}
      mask prompts: alfa "Constante de filtrado"; x0 "Condición inicial"; ts "Período de muestreo"
  Paso a grados : Gain  Gain=GpT
  Paso a rad/s : Gain  Gain=pi/180
  w (rad/s) : Outport
  wires:
  Derivada discreta/1(sal) -> w (rad/s)/1
  Filtro digital paso bajo/1(sal) -> Derivada discreta/1(ent)
  Paso a rad/s/1 -> Filtro digital paso bajo/1(ent)
  Paso a grados/1 -> Paso a rad/s/1
  contador/1 -> Paso a grados/1

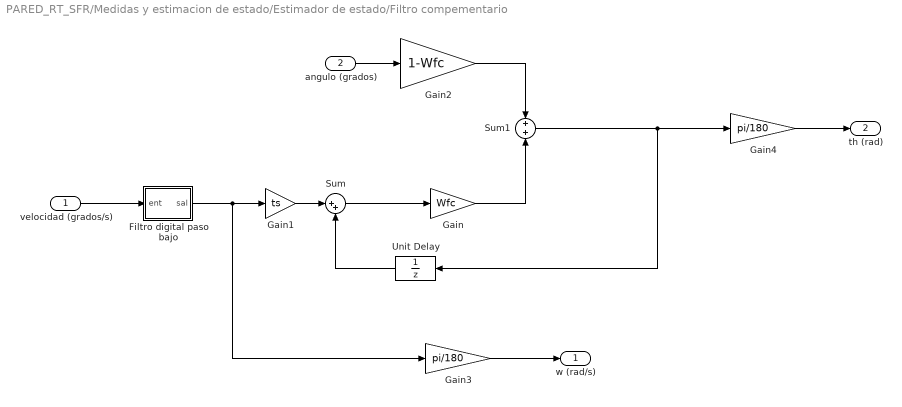
== system PARED_RT_SFR/Medidas y estimacion de estado/Estimador de estado/Filtro compementario ==
  velocidad (grados/s) : Inport  SampleTime=ts
  angulo (grados) : Inport  Port=2  SampleTime=ts
  Filtro digital paso bajo : Subsystem  mask{alfa=alfa1, x0=0, ts=ts}
      mask prompts: alfa "Constante de filtrado"; x0 "Condición inicial"; ts "Período de muestreo"
  Gain : Gain  Gain=Wfc
  Gain1 : Gain  Gain=ts
  Gain2 : Gain  Gain=1-Wfc
  Gain3 : Gain  Gain=pi/180
  Gain4 : Gain  Gain=pi/180
  Sum : Sum  Inputs=|++
  Sum1 : Sum  Inputs=+|+
  Unit Delay : UnitDelay  SampleTime=-1
  w (rad/s) : Outport
  th (rad) : Outport  Port=2
  wires:
  Gain1/1 -> Sum/1
  Unit Delay/1 -> Sum/2
  Sum/1 -> Gain/1
  Gain/1 -> Sum1/2
  angulo (grados)/1 -> Gain2/1
  Gain2/1 -> Sum1/1
  Sum1/1 -> Gain4/1, Unit Delay/1
  Gain3/1 -> w (rad/s)/1
  Gain4/1 -> th (rad)/1
  velocidad (grados/s)/1 -> Filtro digital paso bajo/1(ent)
  Filtro digital paso bajo/1(sal) -> Gain3/1, Gain1/1

== system PARED_RT_SFR/Medidas y estimacion de estado/Estimador de estado/Calculo de la velocidad a partir del contador del encoder/Derivada discreta ==
  ent : Inport  SampleTime=ts
  Discrete Transfer Fcn : DiscreteTransferFcn  Numerator=derivada.num{1}  Denominator=derivada.den{1}
  sal : Outport
  wires:
  ent/1 -> Discrete Transfer Fcn/1
  Discrete Transfer Fcn/1 -> sal/1

== system PARED_RT_SFR/Medidas y estimacion de estado/Estimador de estado/Calculo de la velocidad a partir del contador del encoder/Filtro digital paso bajo ==
  note: Función de transferencia del filtro
      |                        1-alfa
      |                  ----------------
      |                   1-alfa*z^(-1)
  ent : Inport  SampleTime=ts
  Gain2 : Gain  Gain=alfa  OutDataTypeStr=Inherit: Same as input  ParamDataTypeStr=Inherit: Same as input
  Gain3 : Gain  Gain=1-alfa  OutDataTypeStr=Inherit: Same as input  ParamDataTypeStr=Inherit: Same as input
  Sum : Sum  Inputs=|++  OutDataTypeStr=Inherit: Same as first input
  Unit Delay : UnitDelay  SampleTime=-1
  sal : Outport
  wires:
  ent/1 -> Gain3/1
  Gain3/1 -> Sum/1
  Gain2/1 -> Sum/2
  Unit Delay/1 -> Gain2/1
  Sum/1 -> sal/1, Unit Delay/1

== system PARED_RT_SFR/Medidas y estimacion de estado/Estimador de estado/Calculo de la velocidad a partir del contador del encoder /Derivada discreta ==
  ent : Inport  SampleTime=ts
  Discrete Transfer Fcn : DiscreteTransferFcn  Numerator=derivada.num{1}  Denominator=derivada.den{1}
  sal : Outport
  wires:
  Discrete Transfer Fcn/1 -> sal/1
  ent/1 -> Discrete Transfer Fcn/1

== system PARED_RT_SFR/Medidas y estimacion de estado/Estimador de estado/Calculo de la velocidad a partir del contador del encoder /Filtro digital paso bajo ==
  note: Función de transferencia del filtro
      |                        1-alfa
      |                  ----------------
      |                   1-alfa*z^(-1)
  ent : Inport  SampleTime=ts
  Gain2 : Gain  Gain=alfa  OutDataTypeStr=Inherit: Same as input  ParamDataTypeStr=Inherit: Same as input
  Gain3 : Gain  Gain=1-alfa  OutDataTypeStr=Inherit: Same as input  ParamDataTypeStr=Inherit: Same as input
  Sum : Sum  Inputs=|++  OutDataTypeStr=Inherit: Same as first input
  Unit Delay : UnitDelay  SampleTime=-1
  sal : Outport
  wires:
  Sum/1 -> Unit Delay/1, sal/1
  Unit Delay/1 -> Gain2/1
  Gain2/1 -> Sum/2
  Gain3/1 -> Sum/1
  ent/1 -> Gain3/1

== system PARED_RT_SFR/Medidas y estimacion de estado/Estimador de estado/Filtro compementario/Filtro digital paso bajo ==
  note: Función de transferencia del filtro
      |                        1-alfa
      |                  ----------------
      |                   1-alfa*z^(-1)
  ent : Inport  SampleTime=ts
  Gain2 : Gain  Gain=alfa  OutDataTypeStr=Inherit: Same as input  ParamDataTypeStr=Inherit: Same as input
  Gain3 : Gain  Gain=1-alfa  OutDataTypeStr=Inherit: Same as input  ParamDataTypeStr=Inherit: Same as input
  Sum : Sum  Inputs=|++  OutDataTypeStr=Inherit: Same as first input
  Unit Delay : UnitDelay  SampleTime=-1
  sal : Outport
  wires:
  Sum/1 -> Unit Delay/1, sal/1
  Unit Delay/1 -> Gain2/1
  Gain2/1 -> Sum/2
  Gain3/1 -> Sum/1
  ent/1 -> Gain3/1
